simulink subsystem "model_bus_init"  (R2022b)
settings: Solver=VariableStepAuto  StartTime=0.0  StopTime=10.0  RelTol=1e-3
undefined symbols (not defined in the file): d_f_states, d_I_n, d_Ki_id, d_Ki_iq, d_Ki_n, d_Kp_id, d_Kp_iq, d_Kp_n, d_L_d, d_L_q, d_M_n, d_n_n, d_p, d_psi_pm, d_R_ph
settings Model: Creator=valen  LastModifiedBy=valen

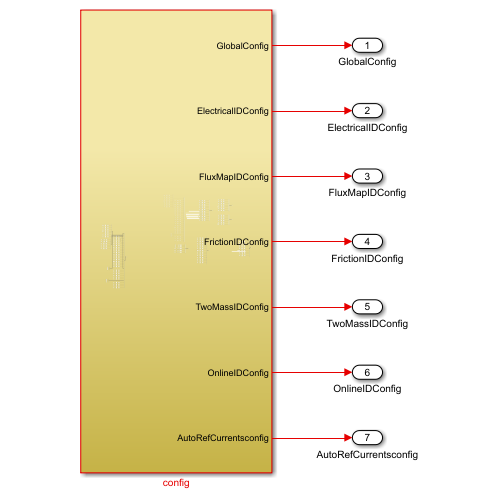
[thumbnail: Simulink's stored preview of the top-level diagram]
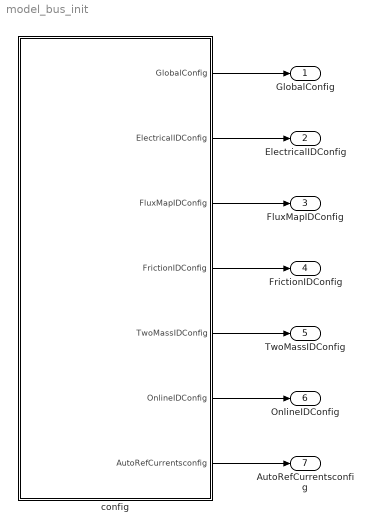
== system model_bus_init ==
  config : Subsystem
  GlobalConfig : Outport
  ElectricalIDConfig : Outport  Port=2
  FluxMapIDConfig : Outport  Port=3
  FrictionIDConfig : Outport  Port=4
  TwoMassIDConfig : Outport  Port=5
  OnlineIDConfig : Outport  Port=6
  AutoRefCurrentsconfig : Outport  Port=7
  wires:
  config/3(FluxMapIDConfig) -> FluxMapIDConfig/1
  config/2(ElectricalIDConfig) -> ElectricalIDConfig/1
  config/1(GlobalConfig) -> GlobalConfig/1
  config/4(FrictionIDConfig) -> FrictionIDConfig/1
  config/5(TwoMassIDConfig) -> TwoMassIDConfig/1
  config/6(OnlineIDConfig) -> OnlineIDConfig/1
  config/7(AutoRefCurrentsconfig) -> AutoRefCurrentsconfig/1

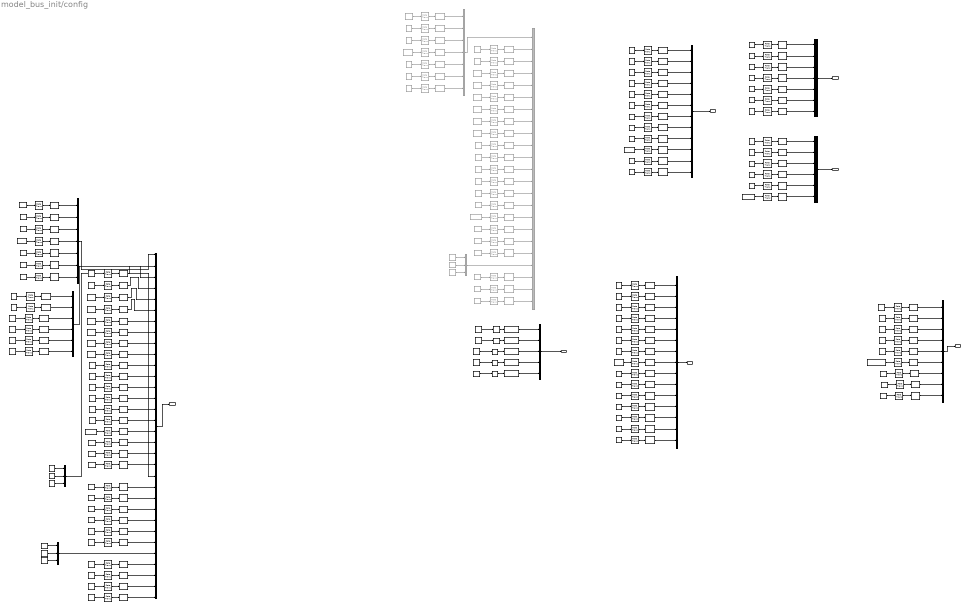
== system model_bus_init/config ==
  note: %1000
  note: Factor for rated speed,to determine the upper end in which interval the linear Parameters will
      | be measured. i.e. 0,5*d_n_n.
      | Default ist 0.625 for 2000rpm
  note: 0: Flux maps will only be calculated, if linear parameters have been identified inside the valid range.
      |     Flux maps will only be calculated again, if the machine is in the valid range.
      | 1:Flux maps will always be calculated, even if the linear parameters were identified outside of range.
  note: Enter value in seconds. Determines, after which time the linear Parameters have to be identified again.
  note: Factor for rated current,to determine in which interval the linear Parameters will
      | be measured. i.e. 0,5*d_I_n
  note: Factor for rated speed,to determine the lower end in which interval the linear Parameters will
      | be measured. i.e. 0,5*d_n_n.
      | Default ist 0.026875 for 86rpm (one rotation during measuring period)
  note: Factor for rated speed,which states when the rotor is rotating fast enough during the DutyCycle evaluation
      | Default ist 0.026875 for 86rpm
  0 = Lq=Ld 1 = identify Lq 1 : Constant
  0 = off 1 = ident R_s online : Constant
  1 : Constant  Commented=on  Value=0.0
  1 = reset : Constant  Commented=on  Value=0
  1 = reset1 : Constant  Value=0
  2 : Constant  Value=0.0
  3 : Constant  Value=0.0
  852 : Constant  Commented=on  Value=0.0
  Activate ControlReference : Constant  OutDataTypeStr=boolean
  Amplitude for SquareWave signal in d-current2 : Constant  Value=0.2
  AutoRefCurrentsConfig_Buscreator : BusCreator  Inputs=5  OutDataTypeStr=Bus: uz_ParaID_AutoRefCurrentsConfig_t
  Bus Creator : BusCreator  Commented=on  Inputs=7  OutDataTypeStr=Bus: uz_PMSM_t
  Bus Creator1 : BusCreator  Inputs=6
  Bus Creator2 : BusCreator  Inputs=7  OutDataTypeStr=Bus: uz_PMSM_t
  Bus Creator3 : BusCreator  Inputs=3  OutDataTypeStr=Bus: uz_3ph_dq_t
  Bus Creator4 : BusCreator  Commented=on  Inputs=3  OutDataTypeStr=Bus: uz_3ph_dq_t
  Bus Creator5 : BusCreator  Inputs=3  OutDataTypeStr=Bus: uz_3ph_dq_t
  C : Constant  Value=0
  Cast To Single : DataTypeConversion  OutDataTypeStr=single  SaturateOnIntegerOverflow=off  RndMeth=Floor
  Cast To Single1 : DataTypeConversion  OutDataTypeStr=single  SaturateOnIntegerOverflow=off  RndMeth=Floor
  Cast To Single2 : DataTypeConversion  OutDataTypeStr=single  SaturateOnIntegerOverflow=off  RndMeth=Floor
  Cast To Single3 : DataTypeConversion  OutDataTypeStr=boolean  SaturateOnIntegerOverflow=off  RndMeth=Floor
  Cast To Single4 : DataTypeConversion  OutDataTypeStr=boolean  SaturateOnIntegerOverflow=off  RndMeth=Floor
  Const{1,47,78,81,91} (5 alike) : Constant  Value=2
  Const{10..11,58,83,94} (5 alike) : Constant  Value=0
  Const12 : Constant  Commented=on  Value=d_M_n
  Const13 : Constant  Value=d_psi_pm
  Const14 : Constant  Value=d_I_n
  Const15 : Constant  Commented=on  Value=d_psi_pm
  Const16 : Constant  Value=d_n_n
  Const17 : Constant  Value=d_L_d
  Const18 : Constant  Value=d_Kp_id
  Const19 : Constant  Value=d_Kp_iq
  Const2 : Constant  Value=5
  Const20 : Constant  Value=d_M_n
  Const21 : Constant  Value=d_Ki_iq
  Const22 : Constant  Value=d_Ki_id
  Const23 : Constant  Value=d_Kp_n
  Const24 : Constant  Value=d_Ki_n
  Const25 : Constant  Value=d_L_q
  Const26 : Constant  Value=d_R_ph
  Const{4,27..28,60,84} (5 alike) : Constant
  Const29 : Constant  Value=0.026875
  Const3 : Constant  Value=0.001
  Const36 : Constant  Commented=on  Value=d_I_n
  Const37 : Constant  Value=20
  Const43 : Constant  Value=0.05
  Const44 : Constant  Value=0.05
  Const5 : Constant  Value=0.077
  Const56 : Constant  Value=0.5
  Const57 : Constant  Value=20
  Const59 : Constant  Value=0.026875
  Const6 : Constant  Value=22
  Const61 : Constant  Commented=on  Value=d_n_n
  Const64 : Constant  Value=0.2
  Const65 : Constant  Value=200
  Const67 : Constant  Value=20
  Const69 : Constant  Value=15
  Const7 : Constant  Commented=on  Value=d_L_d
  Const70 : Constant  Commented=on  Value=d_Kp_id
  Const71 : Constant  Commented=on  Value=d_Kp_iq
  Const73 : Constant  Commented=on  Value=d_Ki_iq
  Const74 : Constant  Commented=on  Value=d_Ki_id
  Const75 : Constant  Commented=on  Value=d_Kp_n
  Const76 : Constant  Commented=on  Value=d_Ki_n
  Const8 : Constant  Commented=on  Value=d_L_q
  Const80 : Constant  Value=-2
  Const82 : Constant  Value=0.0
  Const9 : Constant  Commented=on  Value=d_R_ph
  Const92 : Constant  Value=50
  Const93 : Constant  Value=400
  Const95 : Constant  Value=1/d_f_states
  Constant : Constant  Value=10
  Constant1 : Constant
  Constant2 : Constant  Commented=on
  Constant3 : Constant  Value=20
  Constant4 : Constant  Value=20
  Data Type Conversion{1..2,4,17,52,84,103,136..137} (9 alike) : DataTypeConversion  OutDataTypeStr=uint16  SaturateOnIntegerOverflow=off  RndMeth=Floor
  Data Type Conversion{10..11,23,26,42,51,53,55,59..61,66..67,72,75,78,85..86,93,138} (20 alike) : DataTypeConversion  OutDataTypeStr=boolean  SaturateOnIntegerOverflow=off  RndMeth=Floor
  Data Type Conversion{3,5..9,14,33..41,43..50,54,56..58,62..65,68,70..71,73..74,76..77,79..83,87,91..92,94..95,99..100,105,118,120..124,134..135,139} (61 alike) : DataTypeConversion  OutDataTypeStr=single  SaturateOnIntegerOverflow=off  RndMeth=Floor
  Data Type Conversion{16,21..22,31..32,109,144..145} (8 alike) : DataTypeConversion  Commented=on  OutDataTypeStr=boolean  SaturateOnIntegerOverflow=off  RndMeth=Floor
  Data Type Conversion{12..13,15,18..20,25,27..30,69,96,110..115} (19 alike) : DataTypeConversion  Commented=on  OutDataTypeStr=single  SaturateOnIntegerOverflow=off  RndMeth=Floor
  Data Type Conversion24 : DataTypeConversion  Commented=on  OutDataTypeStr=uint16  SaturateOnIntegerOverflow=off  RndMeth=Floor
  ElectricalIDConfig_Buscreater1 : BusCreator  Inputs=9  OutDataTypeStr=Bus: uz_ParaID_ElectricalIDConfig_t
  Enable output : Constant
  FluxMapIDConfig_Buscreater : BusCreator  Inputs=15  OutDataTypeStr=Bus: uz_ParaID_FluxMapIDConfig_t
  FrictionIDConfig_Buscreater : BusCreator  Inputs=7  OutDataTypeStr=Bus: uz_ParaID_FrictionIDConfig_t
  GlobalConfig_Buscreator : BusCreator  Commented=on  Inputs=23  OutDataTypeStr=Bus: uz_ParaID_GlobalConfig_t
  GlobalConfig_Buscreator1 : BusCreator  Inputs=32  OutDataTypeStr=Bus: uz_ParaID_GlobalConfig_t
  ISR sample time 0.1 : Constant  Commented=on  Value=1/d_f_states
  ISR sample time 0.2 : Constant  Value=1/d_f_states
  M_ref : Constant  Commented=on  Value=0
  M_ref1 : Constant  Value=0
  Number of pole pairs1 : Constant  Value=d_p
  Number of pole pairs2 : Constant  Commented=on  Value=d_p
  OnlineIDConfig_Buscreater : BusCreator  Inputs=12  OutDataTypeStr=Bus: uz_ParaID_OnlineIDConfig_t
  PI_subs : Constant  Value=0
  Rate Transition{1..12,18,23..24,26,33..35,37..64,66..92,94..98,116..117,120,122,169,171..175,217..222} (95 alike) : RateTransition  OutPortSampleTime=1/d_f_states
  Rate Transition{13..17,19..22,25,27..32,36,65,99,102..103,148..154} (28 alike) : RateTransition  Commented=on  OutPortSampleTime=1/d_f_states
  Reset ControlReference : Constant  Value=0  OutDataTypeStr=boolean
  Rp : Constant  Value=0
  Rs : Constant  Value=0
  TwoMassIDConfig_Buscreater : BusCreator  Inputs=6  OutDataTypeStr=Bus: uz_ParaID_TwoMassIDConfig_t
  controllers_updated : Constant  Value=0
  doElectricalID : Constant  Commented=on
  doElectricalID1 : Constant
  doFluxMapID : Constant  Commented=on  Value=0
  doFluxMapID1 : Constant  Value=0
  doFrictionID : Constant  Commented=on  Value=0
  doFrictionID1 : Constant  Value=0
  doTwoMassID : Constant  Commented=on
  doTwoMassID1 : Constant  Value=0
  enableOnlineID : Constant  Commented=on  Value=0
  enableOnlineID1 : Constant  Value=0
  enableParameterID : Constant  Commented=on
  enableParameterID{1..7} (7 alike) : Constant
  extended_offset 3 : Constant
  extended_psi : Constant
  goertzlFreq in Hz1 : Constant  Value=40
  i_d : Constant  Commented=on  Value=0  OutDataTypeStr=single
  i_d1 : Constant  Value=0  OutDataTypeStr=single
  i_d3 : Constant  Value=0  OutDataTypeStr=single
  i_q : Constant  Commented=on  Value=0  OutDataTypeStr=single
  i_q1 : Constant  Value=0  OutDataTypeStr=single
  i_q3 : Constant  Value=0  OutDataTypeStr=single
  i_zero : Constant  Commented=on  Value=0  OutDataTypeStr=single
  i_zero1 : Constant  Value=0  OutDataTypeStr=single
  i_zero3 : Constant  Value=0  OutDataTypeStr=single
  manual input of a DutyCycle1 : Constant  Value=0.5
  manual_offset : Constant
  motor_type : Constant  Commented=on  Value=0
  motor_type1 : Constant  Value=0
  n_ref : Constant  Commented=on  Value=0
  n_ref measurement1 : Constant  Value=400
  n_ref measurement2 : Constant  Value=500
  n_ref1 : Constant  Value=0
  res_subs : Constant  Value=0
  selected_subs : Constant
  setpoint_filter : Constant  Value=0
  temp_ll : Constant
  temp_ul : Constant
  GlobalConfig : Outport
  ElectricalIDConfig : Outport  Port=2
  FluxMapIDConfig : Outport  Port=3
  FrictionIDConfig : Outport  Port=4
  TwoMassIDConfig : Outport  Port=5
  OnlineIDConfig : Outport  Port=6
  AutoRefCurrentsconfig : Outport  Port=7
  wires:
  Data Type Conversion1/1 -> FrictionIDConfig_Buscreater/2  "N_Brk"
  Data Type Conversion99/1 -> FrictionIDConfig_Buscreater/6  "eta"
  Data Type Conversion2/1 -> FrictionIDConfig_Buscreater/3  "N_Visco"
  Data Type Conversion103/1 -> FrictionIDConfig_Buscreater/1  "BrkCount"
  Data Type Conversion105/1 -> FrictionIDConfig_Buscreater/7  "maxCurrent"
  Data Type Conversion100/1 -> FrictionIDConfig_Buscreater/5  "n_eva_max"
  Data Type Conversion3/1 -> FrictionIDConfig_Buscreater/4  "StepScale"
  FrictionIDConfig_Buscreater/1 -> FrictionIDConfig/1
  Rate Transition120/1 -> Data Type Conversion103/1
  Const67/1 -> Rate Transition120/1
  Const1/1 -> Rate Transition1/1
  Rate Transition1/1 -> Data Type Conversion1/1
  Const2/1 -> Rate Transition2/1
  Rate Transition2/1 -> Data Type Conversion2/1
  Const3/1 -> Rate Transition3/1
  Rate Transition3/1 -> Data Type Conversion3/1
  Const65/1 -> Rate Transition117/1
  Const64/1 -> Rate Transition116/1
  Rate Transition116/1 -> Data Type Conversion99/1
  Rate Transition117/1 -> Data Type Conversion100/1
  Const69/1 -> Rate Transition122/1
  Rate Transition122/1 -> Data Type Conversion105/1
  TwoMassIDConfig_Buscreater/1 -> TwoMassIDConfig/1
  Const91/1 -> Rate Transition217/1
  Rate Transition217/1 -> Data Type Conversion134/1
  Data Type Conversion134/1 -> TwoMassIDConfig_Buscreater/1  "ScaleTorquePRBS"
  Rate Transition218/1 -> Data Type Conversion135/1
  n_ref measurement1/1 -> Rate Transition218/1
  Data Type Conversion135/1 -> TwoMassIDConfig_Buscreater/2  "n_ref_measurement"
  Rate Transition219/1 -> Data Type Conversion136/1
  Const93/1 -> Rate Transition220/1
  Const92/1 -> Rate Transition219/1
  Rate Transition220/1 -> Data Type Conversion137/1
  Data Type Conversion137/1 -> TwoMassIDConfig_Buscreater/3  "f_max"
  Data Type Conversion136/1 -> TwoMassIDConfig_Buscreater/4  "f_min"
  Rate Transition221/1 -> Data Type Conversion138/1
  Rate Transition222/1 -> Data Type Conversion139/1
  Const94/1 -> Rate Transition221/1
  Const95/1 -> Rate Transition222/1
  Data Type Conversion138/1 -> TwoMassIDConfig_Buscreater/5  "UseLbMq"
  Data Type Conversion139/1 -> TwoMassIDConfig_Buscreater/6  "d_TMS_start"
  OnlineIDConfig_Buscreater/1 -> OnlineIDConfig/1
  Const37/1 -> Rate Transition52/1
  Rate Transition52/1 -> Data Type Conversion56/1
  Data Type Conversion56/1 -> OnlineIDConfig_Buscreater/2  "Temp_ref"
  Data Type Conversion77/1 -> OnlineIDConfig_Buscreater/4  "dev_curr"
  Data Type Conversion76/1 -> OnlineIDConfig_Buscreater/3  "dev_omega"
  Const44/1 -> Rate Transition73/1
  Const43/1 -> Rate Transition72/1
  Rate Transition72/1 -> Data Type Conversion76/1
  Const47/1 -> Rate Transition76/1
  Rate Transition73/1 -> Data Type Conversion77/1
  Rate Transition76/1 -> Data Type Conversion80/1
  Data Type Conversion80/1 -> OnlineIDConfig_Buscreater/5  "identRAmp"
  Data Type Conversion61/1 -> OnlineIDConfig_Buscreater/6  "AverageTransParams"
  Const28/1 -> Rate Transition79/1
  Rate Transition79/1 -> Data Type Conversion61/1
  Const56/1 -> Rate Transition94/1
  Data Type Conversion93/1 -> OnlineIDConfig_Buscreater/9  "allowPsiCalcOutside"
  Rate Transition94/1 -> Data Type Conversion91/1
  Data Type Conversion95/1 -> OnlineIDConfig_Buscreater/11  "max_n_ratio"
  Const58/1 -> Rate Transition96/1
  Const57/1 -> Rate Transition95/1
  Data Type Conversion91/1 -> OnlineIDConfig_Buscreater/7  "nom_factor"
  Rate Transition98/1 -> Data Type Conversion95/1
  Data Type Conversion92/1 -> OnlineIDConfig_Buscreater/8  "Rs_time"
  Rate Transition96/1 -> Data Type Conversion93/1
  Const59/1 -> Rate Transition97/1
  Rate Transition97/1 -> Data Type Conversion94/1
  Const60/1 -> Rate Transition98/1
  Data Type Conversion94/1 -> OnlineIDConfig_Buscreater/10  "min_n_ratio"
  Rate Transition95/1 -> Data Type Conversion92/1
  1 = reset/1 -> Rate Transition148/1
  Rate Transition149/1 -> Data Type Conversion110/1
  Const75/1 -> Rate Transition153/1
  Rate Transition150/1 -> Data Type Conversion111/1
  Rate Transition152/1 -> Data Type Conversion113/1
  Const71/1 -> Rate Transition150/1
  Rate Transition154/1 -> Data Type Conversion115/1
  Const76/1 -> Rate Transition154/1
  Rate Transition148/1 -> Data Type Conversion109/1
  Const70/1 -> Rate Transition149/1
  Rate Transition153/1 -> Data Type Conversion114/1
  Const73/1 -> Rate Transition151/1
  Rate Transition151/1 -> Data Type Conversion112/1
  Const74/1 -> Rate Transition152/1
  Data Type Conversion109/1 -> GlobalConfig_Buscreator/3  "Reset"
  Data Type Conversion110/1 -> GlobalConfig_Buscreator/4  "Kp_id"
  Data Type Conversion111/1 -> GlobalConfig_Buscreator/5  "Kp_iq"
  Data Type Conversion114/1 -> GlobalConfig_Buscreator/6  "Kp_n"
  Data Type Conversion113/1 -> GlobalConfig_Buscreator/7  "Ki_id"
  Data Type Conversion112/1 -> GlobalConfig_Buscreator/8  "Ki_iq"
  Data Type Conversion115/1 -> GlobalConfig_Buscreator/9  "Ki_n"
  Rate Transition28/1 -> Data Type Conversion31/1
  Data Type Conversion32/1 -> GlobalConfig_Buscreator/11  "FrictionID"
  doTwoMassID/1 -> Rate Transition102/1
  Data Type Conversion145/1 -> GlobalConfig_Buscreator/13  "FluxMapID"
  Rate Transition29/1 -> Data Type Conversion32/1
  doFluxMapID/1 -> Rate Transition103/1
  Rate Transition103/1 -> Data Type Conversion145/1
  Data Type Conversion31/1 -> GlobalConfig_Buscreator/10  "ElectricalID"
  Rate Transition102/1 -> Data Type Conversion144/1
  doElectricalID/1 -> Rate Transition28/1
  Data Type Conversion144/1 -> GlobalConfig_Buscreator/12  "TwoMassID"
  doFrictionID/1 -> Rate Transition29/1
  Constant2/1 -> Rate Transition16/1
  Rate Transition16/1 -> Data Type Conversion16/1
  Data Type Conversion16/1 -> GlobalConfig_Buscreator/15  "ACCEPT"
  ISR sample time 0.1/1 -> Rate Transition20/1
  Rate Transition20/1 -> Data Type Conversion20/1
  Const36/1 -> Rate Transition65/1
  Const61/1 -> Rate Transition99/1
  Rate Transition99/1 -> Data Type Conversion96/1
  Rate Transition65/1 -> Data Type Conversion69/1
  Data Type Conversion69/1 -> GlobalConfig_Buscreator/17  "ratCurrent"
  Data Type Conversion96/1 -> GlobalConfig_Buscreator/19  "ratSpeed"
  enableOnlineID/1 -> Rate Transition21/1
  Data Type Conversion21/1 -> GlobalConfig_Buscreator/14  "OnlineID"
  Rate Transition21/1 -> Data Type Conversion21/1
  Rate Transition26/1 -> Data Type Conversion26/1
  Data Type Conversion26/1 -> OnlineIDConfig_Buscreater/1  "OnlineID_Reset"
  Const10/1 -> Rate Transition26/1
  Bus Creator/1 -> GlobalConfig_Buscreator/1  "PMSM_config"
  Const15/1 -> Rate Transition15/1
  Rate Transition15/1 -> Data Type Conversion15/1
  Data Type Conversion15/1 -> Bus Creator/4  "Psi_PM_Vs"
  Rate Transition30/1 -> Data Type Conversion28/1
  Number of pole pairs2/1 -> Rate Transition30/1
  Data Type Conversion28/1 -> Bus Creator/5  "polePairs"
  Rate Transition31/1 -> Data Type Conversion29/1
  852/1 -> Rate Transition31/1
  Data Type Conversion29/1 -> Bus Creator/6  "J_kg_m_squared"
  Rate Transition32/1 -> Data Type Conversion30/1
  1/1 -> Rate Transition32/1
  Data Type Conversion30/1 -> Bus Creator/7  "I_max_Ampere"
  Data Type Conversion13/1 -> Bus Creator/1  "R_ph_Ohm"
  Const9/1 -> Rate Transition14/1
  Rate Transition14/1 -> Data Type Conversion13/1
  Data Type Conversion27/1 -> Bus Creator/2  "Ld_Henry"
  Rate Transition13/1 -> Data Type Conversion12/1
  Rate Transition27/1 -> Data Type Conversion27/1
  Data Type Conversion12/1 -> Bus Creator/3  "Lq_Henry"
  Const7/1 -> Rate Transition27/1
  Const8/1 -> Rate Transition13/1
  i_q/1 -> Bus Creator4/2  "q"
  i_d/1 -> Bus Creator4/1  "d"
  i_zero/1 -> Bus Creator4/3  "zero"
  Bus Creator4/1 -> GlobalConfig_Buscreator/20  "i_dq_ref"
  Rate Transition19/1 -> Data Type Conversion19/1
  n_ref/1 -> Rate Transition19/1
  Data Type Conversion19/1 -> GlobalConfig_Buscreator/21  "n_ref"
  enableParameterID/1 -> Rate Transition22/1
  Rate Transition22/1 -> Data Type Conversion22/1
  Data Type Conversion22/1 -> GlobalConfig_Buscreator/2  "enableParameterID"
  Rate Transition23/1 -> Data Type Conversion23/1
  Const11/1 -> Rate Transition23/1
  Data Type Conversion23/1 -> OnlineIDConfig_Buscreater/12  "array_cleaned"
  Constant4/1 -> Rate Transition88/1
  Rate Transition88/1 -> Cast To Single/1
  Rate Transition24/1 -> Cast To Single1/1
  Constant3/1 -> Rate Transition24/1
  Rate Transition33/1 -> Cast To Single2/1
  Constant/1 -> Rate Transition33/1
  Rate Transition34/1 -> Cast To Single3/1
  Cast To Single3/1 -> AutoRefCurrentsConfig_Buscreator/1  "enableCRS"
  Activate ControlReference/1 -> Rate Transition34/1
  Rate Transition35/1 -> Cast To Single4/1
  Reset ControlReference/1 -> Rate Transition35/1
  Cast To Single4/1 -> AutoRefCurrentsConfig_Buscreator/2  "Reset"
  Cast To Single/1 -> AutoRefCurrentsConfig_Buscreator/3  "iq_points"
  Cast To Single1/1 -> AutoRefCurrentsConfig_Buscreator/4  "id_points"
  Cast To Single2/1 -> AutoRefCurrentsConfig_Buscreator/5  "max_current"
  AutoRefCurrentsConfig_Buscreator/1 -> AutoRefCurrentsconfig/1
  Data Type Conversion20/1 -> GlobalConfig_Buscreator/16  "sampleTimeISR"
  Rate Transition17/1 -> Data Type Conversion18/1
  Const12/1 -> Rate Transition17/1
  Data Type Conversion18/1 -> GlobalConfig_Buscreator/18  "ratTorque"
  motor_type/1 -> Rate Transition25/1
  Rate Transition25/1 -> Data Type Conversion24/1
  Data Type Conversion24/1 -> GlobalConfig_Buscreator/23  "motor_type"
  M_ref/1 -> Rate Transition36/1
  Rate Transition36/1 -> Data Type Conversion25/1
  Data Type Conversion25/1 -> GlobalConfig_Buscreator/22  "M_ref"
  i_d3/1 -> Bus Creator5/1  "d"
  Data Type Conversion35/1 -> GlobalConfig_Buscreator1/27  "voltage_measurement_Rs"
  Rate Transition43/1 -> Data Type Conversion39/1
  enableParameterID4/1 -> Rate Transition42/1
  Bus Creator5/1 -> GlobalConfig_Buscreator1/28  "i_xy_ref"
  Bus Creator2/1 -> GlobalConfig_Buscreator1/1  "PMSM_config"
  i_q3/1 -> Bus Creator5/2  "q"
  Data Type Conversion66/1 -> GlobalConfig_Buscreator1/11  "ElectricalID"
  enableParameterID5/1 -> Rate Transition43/1
  Data Type Conversion33/1 -> GlobalConfig_Buscreator1/25  "voltage_measurement_C"
  Data Type Conversion60/1 -> GlobalConfig_Buscreator1/3  "enableParameterID"
  Data Type Conversion38/1 -> Bus Creator1/3  "x"
  Rate Transition71/1 -> Data Type Conversion65/1
  Rate Transition74/1 -> Data Type Conversion68/1
  doFrictionID1/1 -> Rate Transition68/1
  enableParameterID6/1 -> Rate Transition44/1
  i_zero3/1 -> Bus Creator5/3  "zero"
  enableParameterID7/1 -> Rate Transition45/1
  Rs/1 -> Rate Transition39/1
  Data Type Conversion44/1 -> GlobalConfig_Buscreator1/6  "Kp_iq"
  Rate Transition40/1 -> Data Type Conversion36/1
  Rate Transition60/1 -> Data Type Conversion55/1
  Data Type Conversion34/1 -> GlobalConfig_Buscreator1/26  "voltage_measurement_Rp"
  Const18/1 -> Rate Transition53/1
  Data Type Conversion51/1 -> GlobalConfig_Buscreator1/13  "TwoMassID"
  Rate Transition49/1 -> Data Type Conversion49/1
  Rate Transition66/1 -> Data Type Conversion62/1
  Data Type Conversion59/1 -> GlobalConfig_Buscreator1/15  "OnlineID"
  i_q1/1 -> Bus Creator3/2  "q"
  Data Type Conversion47/1 -> GlobalConfig_Buscreator1/7  "Kp_n"
  Const26/1 -> Rate Transition50/1
  Data Type Conversion40/1 -> Bus Creator1/5  "z1"
  Rate Transition50/1 -> Data Type Conversion50/1
  Rate Transition55/1 -> Data Type Conversion44/1
  Data Type Conversion39/1 -> Bus Creator1/4  "y"
  Rate Transition45/1 -> Data Type Conversion41/1
  Rate Transition42/1 -> Data Type Conversion38/1
  Data Type Conversion37/1 -> Bus Creator1/2  "q"
  Rate Transition41/1 -> Data Type Conversion37/1
  Data Type Conversion70/1 -> GlobalConfig_Buscreator1/20  "ratSpeed"
  Data Type Conversion43/1 -> GlobalConfig_Buscreator1/5  "Kp_id"
  enableOnlineID1/1 -> Rate Transition63/1
  Rate Transition53/1 -> Data Type Conversion43/1
  1 = reset1/1 -> Rate Transition51/1
  Bus Creator1/1 -> GlobalConfig_Buscreator1/2  "PMSM_6ph_inductances"
  i_zero1/1 -> Bus Creator3/3  "zero"
  Rp/1 -> Rate Transition38/1
  Rate Transition37/1 -> Data Type Conversion33/1
  enableParameterID3/1 -> Rate Transition41/1
  n_ref1/1 -> Rate Transition61/1
  doFluxMapID1/1 -> Rate Transition47/1
  Constant1/1 -> Rate Transition60/1
  Rate Transition57/1 -> Data Type Conversion46/1
  Const19/1 -> Rate Transition55/1
  Data Type Conversion64/1 -> Bus Creator2/6  "J_kg_m_squared"
  Data Type Conversion50/1 -> Bus Creator2/1  "R_ph_Ohm"
  Data Type Conversion63/1 -> Bus Creator2/5  "polePairs"
  Data Type Conversion62/1 -> Bus Creator2/2  "Ld_Henry"
  Data Type Conversion58/1 -> GlobalConfig_Buscreator1/17  "sampleTimeISR"
  Data Type Conversion67/1 -> GlobalConfig_Buscreator1/12  "FrictionID"
  Data Type Conversion65/1 -> Bus Creator2/7  "I_max_Ampere"
  Rate Transition47/1 -> Data Type Conversion53/1
  Rate Transition56/1 -> Data Type Conversion45/1
  Number of pole pairs1/1 -> Rate Transition69/1
  Data Type Conversion48/1 -> GlobalConfig_Buscreator1/10  "Ki_n"
  Data Type Conversion46/1 -> GlobalConfig_Buscreator1/8  "Ki_id"
  GlobalConfig_Buscreator1/1 -> GlobalConfig/1
  enableParameterID1/1 -> Rate Transition64/1
  Const16/1 -> Rate Transition75/1
  Const23/1 -> Rate Transition58/1
  Data Type Conversion54/1 -> Bus Creator2/4  "Psi_PM_Vs"
  Data Type Conversion55/1 -> GlobalConfig_Buscreator1/16  "ACCEPT"
  Rate Transition68/1 -> Data Type Conversion67/1
  doElectricalID1/1 -> Rate Transition67/1
  Rate Transition64/1 -> Data Type Conversion60/1
  Rate Transition44/1 -> Data Type Conversion40/1
  Data Type Conversion45/1 -> GlobalConfig_Buscreator1/9  "Ki_iq"
  Rate Transition58/1 -> Data Type Conversion47/1
  Rate Transition38/1 -> Data Type Conversion34/1
  Rate Transition63/1 -> Data Type Conversion59/1
  enableParameterID2/1 -> Rate Transition40/1
  ISR sample time 0.2/1 -> Rate Transition62/1
  Const14/1 -> Rate Transition74/1
  i_d1/1 -> Bus Creator3/1  "d"
  Rate Transition54/1 -> Data Type Conversion54/1
  Rate Transition67/1 -> Data Type Conversion66/1
  Const22/1 -> Rate Transition57/1
  2/1 -> Rate Transition71/1
  C/1 -> Rate Transition37/1
  Const24/1 -> Rate Transition59/1
  Data Type Conversion53/1 -> GlobalConfig_Buscreator1/14  "FluxMapID"
  Data Type Conversion68/1 -> GlobalConfig_Buscreator1/18  "ratCurrent"
  Rate Transition51/1 -> Data Type Conversion42/1
  Rate Transition39/1 -> Data Type Conversion35/1
  3/1 -> Rate Transition70/1
  Rate Transition70/1 -> Data Type Conversion64/1
  Rate Transition59/1 -> Data Type Conversion48/1
  Rate Transition69/1 -> Data Type Conversion63/1
  Rate Transition61/1 -> Data Type Conversion57/1
  Data Type Conversion57/1 -> GlobalConfig_Buscreator1/22  "n_ref"
  Const17/1 -> Rate Transition66/1
  Data Type Conversion42/1 -> GlobalConfig_Buscreator1/4  "Reset"
  Const21/1 -> Rate Transition56/1
  Bus Creator3/1 -> GlobalConfig_Buscreator1/21  "i_dq_ref"
  Const13/1 -> Rate Transition54/1
  Data Type Conversion36/1 -> Bus Creator1/1  "d"
  Const25/1 -> Rate Transition49/1
  Rate Transition75/1 -> Data Type Conversion70/1
  Data Type Conversion49/1 -> Bus Creator2/3  "Lq_Henry"
  doTwoMassID1/1 -> Rate Transition46/1
  Rate Transition46/1 -> Data Type Conversion51/1
  Data Type Conversion41/1 -> Bus Creator1/6  "z2"
  Rate Transition62/1 -> Data Type Conversion58/1
  Data Type Conversion71/1 -> GlobalConfig_Buscreator1/23  "M_ref"
  Rate Transition77/1 -> Data Type Conversion71/1
  M_ref1/1 -> Rate Transition77/1
  extended_offset 3/1 -> Rate Transition83/1
  manual_offset/1 -> Rate Transition84/1
  Rate Transition84/1 -> Data Type Conversion79/1
  extended_psi/1 -> Rate Transition82/1
  Data Type Conversion78/1 -> ElectricalIDConfig_Buscreater1/8  "extended_offset"
  Data Type Conversion79/1 -> ElectricalIDConfig_Buscreater1/9  "manual_offset"
  Data Type Conversion75/1 -> ElectricalIDConfig_Buscreater1/7  "extended_psi"
  Data Type Conversion72/1 -> ElectricalIDConfig_Buscreater1/4  "identLq"
  Const27/1 -> Rate Transition85/1
  Data Type Conversion83/1 -> ElectricalIDConfig_Buscreater1/6  "min_n_ratio"
  Data Type Conversion81/1 -> ElectricalIDConfig_Buscreater1/5  "goertzlTorque"
  0 = Lq=Ld 1 = identify Lq 1/1 -> Rate Transition86/1
  Const29/1 -> Rate Transition78/1
  Rate Transition78/1 -> Data Type Conversion83/1
  Rate Transition85/1 -> Data Type Conversion81/1
  goertzlFreq in Hz1/1 -> Rate Transition81/1
  Data Type Conversion73/1 -> ElectricalIDConfig_Buscreater1/3  "n_ref_measurement"
  Rate Transition82/1 -> Data Type Conversion75/1
  Rate Transition87/1 -> Data Type Conversion82/1
  Rate Transition86/1 -> Data Type Conversion72/1
  Data Type Conversion74/1 -> ElectricalIDConfig_Buscreater1/1  "goertzlFreq"
  Rate Transition83/1 -> Data Type Conversion78/1
  Rate Transition81/1 -> Data Type Conversion74/1
  Data Type Conversion82/1 -> ElectricalIDConfig_Buscreater1/2  "dutyCyc"
  Rate Transition80/1 -> Data Type Conversion73/1
  n_ref measurement2/1 -> Rate Transition80/1
  manual input of a DutyCycle1/1 -> Rate Transition87/1
  ElectricalIDConfig_Buscreater1/1 -> ElectricalIDConfig/1
  Rate Transition9/1 -> Data Type Conversion9/1
  FluxMapIDConfig_Buscreater/1 -> FluxMapIDConfig/1
  Rate Transition12/1 -> Data Type Conversion10/1
  Rate Transition6/1 -> Data Type Conversion6/1
  selected_subs/1 -> Rate Transition4/1
  Rate Transition171/1 -> Data Type Conversion120/1
  Data Type Conversion5/1 -> FluxMapIDConfig_Buscreater/14  "lower_meas_temp"
  Rate Transition173/1 -> Data Type Conversion122/1
  Data Type Conversion123/1 -> FluxMapIDConfig_Buscreater/5  "IQstart"
  Rate Transition169/1 -> Data Type Conversion118/1
  Rate Transition4/1 -> Data Type Conversion4/1
  Rate Transition175/1 -> Data Type Conversion124/1
  Amplitude for SquareWave signal in d-current2/1 -> Rate Transition10/1
  temp_ll/1 -> Rate Transition5/1
  Const4/1 -> Rate Transition7/1
  Const81/1 -> Rate Transition172/1
  Data Type Conversion121/1 -> FluxMapIDConfig_Buscreater/3  "IDstepsize"
  Data Type Conversion118/1 -> FluxMapIDConfig_Buscreater/1  "AMMsampleTime"
  Rate Transition10/1 -> Data Type Conversion14/1
  Const82/1 -> Rate Transition173/1
  Data Type Conversion4/1 -> FluxMapIDConfig_Buscreater/13  "selected_subsystem"
  Data Type Conversion14/1 -> FluxMapIDConfig_Buscreater/12  "identRAmp"
  Rate Transition11/1 -> Data Type Conversion11/1
  Data Type Conversion8/1 -> FluxMapIDConfig_Buscreater/8  "R_s_ref"
  Const6/1 -> Rate Transition9/1
  Const83/1 -> Rate Transition174/1
  Rate Transition8/1 -> Data Type Conversion8/1
  Data Type Conversion11/1 -> FluxMapIDConfig_Buscreater/11  "identR"
  Data Type Conversion124/1 -> FluxMapIDConfig_Buscreater/6  "IQstepsize"
  0 = off 1 = ident R_s online/1 -> Rate Transition11/1
  Data Type Conversion122/1 -> FluxMapIDConfig_Buscreater/4  "IDstop"
  Const5/1 -> Rate Transition8/1
  temp_ul/1 -> Rate Transition6/1
  Data Type Conversion7/1 -> FluxMapIDConfig_Buscreater/7  "IQstop"
  Const78/1 -> Rate Transition169/1
  Data Type Conversion9/1 -> FluxMapIDConfig_Buscreater/9  "Temp_ref"
  Data Type Conversion10/1 -> FluxMapIDConfig_Buscreater/10  "start_FM_ID"
  Rate Transition172/1 -> Data Type Conversion121/1
  Rate Transition5/1 -> Data Type Conversion5/1
  Rate Transition174/1 -> Data Type Conversion123/1
  Data Type Conversion6/1 -> FluxMapIDConfig_Buscreater/15  "upper_meas_temp"
  Const80/1 -> Rate Transition171/1
  Data Type Conversion120/1 -> FluxMapIDConfig_Buscreater/2  "IDstart"
  Enable output/1 -> Rate Transition12/1
  Const84/1 -> Rate Transition175/1
  Rate Transition7/1 -> Data Type Conversion7/1
  motor_type1/1 -> Rate Transition18/1
  Data Type Conversion17/1 -> GlobalConfig_Buscreator1/24  "motor_type"
  Rate Transition18/1 -> Data Type Conversion17/1
  Rate Transition48/1 -> Data Type Conversion52/1
  res_subs/1 -> Rate Transition48/1
  Data Type Conversion52/1 -> GlobalConfig_Buscreator1/29  "resonant_subsystem"
  Data Type Conversion84/1 -> GlobalConfig_Buscreator1/30  "PI_subsystem"
  PI_subs/1 -> Rate Transition89/1
  Rate Transition89/1 -> Data Type Conversion84/1
  Rate Transition90/1 -> Data Type Conversion85/1
  controllers_updated/1 -> Rate Transition90/1
  Data Type Conversion85/1 -> GlobalConfig_Buscreator1/31  "controllers_updated"
  Data Type Conversion86/1 -> GlobalConfig_Buscreator1/32  "setpoint_filter"
  setpoint_filter/1 -> Rate Transition91/1
  Rate Transition91/1 -> Data Type Conversion86/1
  Rate Transition92/1 -> Data Type Conversion87/1
  Data Type Conversion87/1 -> GlobalConfig_Buscreator1/19  "ratTorque"
  Const20/1 -> Rate Transition92/1
